simulink model "BalancingRobot_backup"  (R2020a)
settings: Solver=ode23t  StartTime=0.0  StopTime=20  RelTol=1e-2  EnableMultiTasking=on
values from neighbouring files (symbols this model uses):
  height_plane = 0.01    [DDPG_episdoe_508_maxtorque_2175e-01_Tf_10_Ts_1e-01_6DOF.mat]    (also in DDPG_episode_119_before_6dof_change_Ts_1e-01.mat)
  init_height = 0.109    [DDPG_episdoe_508_maxtorque_2175e-01_Tf_10_Ts_1e-01_6DOF.mat]    (also in DDPG_episode_119_before_6dof_change_Ts_1e-01.mat)
  max_torque = 0.2157463    [DDPG_episdoe_508_maxtorque_2175e-01_Tf_10_Ts_1e-01_6DOF.mat]    (also in DDPG_episode_119_before_6dof_change_Ts_1e-01.mat)
  plane_x = 10    [DDPG_episdoe_508_maxtorque_2175e-01_Tf_10_Ts_1e-01_6DOF.mat]    (also in DDPG_episode_119_before_6dof_change_Ts_1e-01.mat)
  plane_y = 1    [DDPG_episdoe_508_maxtorque_2175e-01_Tf_10_Ts_1e-01_6DOF.mat]    (also in DDPG_episode_119_before_6dof_change_Ts_1e-01.mat)
  table =     [DDPG_episdoe_508_maxtorque_2175e-01_Tf_10_Ts_1e-01_6DOF.mat]    (also in DDPG_episode_119_before_6dof_change_Ts_1e-01.mat)
  Tf = 10    [DDPG_episdoe_508_maxtorque_2175e-01_Tf_10_Ts_1e-01_6DOF.mat]    (also in DDPG_episode_119_before_6dof_change_Ts_1e-01.mat)
  Ts = 0.1    [DDPG_episdoe_508_maxtorque_2175e-01_Tf_10_Ts_1e-01_6DOF.mat]    (also in DDPG_episode_119_before_6dof_change_Ts_1e-01.mat)
  vx0 = 0    [DDPG_episdoe_508_maxtorque_2175e-01_Tf_10_Ts_1e-01_6DOF.mat]    (also in DDPG_episode_119_before_6dof_change_Ts_1e-01.mat)
  whl =     [DDPG_episdoe_508_maxtorque_2175e-01_Tf_10_Ts_1e-01_6DOF.mat]    (also in DDPG_episode_119_before_6dof_change_Ts_1e-01.mat)
undefined symbols (not defined in the file or in its folder): X, Y, Z
libraries: sm_lib x72, nesl_utility x22, Contact_Forces_Lib x14, simulink x8, rllib x1
(part 1 of 4)
settings Model: Creator=The MathWorks, Inc.  LastModifiedBy=User
settings SolverCC: ZeroCrossAlgorithm=Adaptive
settings DataIOCC: SaveOutput=off  SignalLogging=off  DSMLogging=off  SaveTime=off  ReturnWorkspaceOutputs=off  OutputTimes=0:0.01:10
settings OptimizationCC: LifeSpan=inf
settings DebuggingCC: MaxConsecutiveZCsMsg=warning  IgnoredZcDiagnostic=none  AllowSymbolicDim=off  SFUnexpectedBacktrackingDiag=warning  SFNoUnconditionalDefaultTransitionDiag=warning  SFExecutionAtInitializationDiag=none  UnitsInconsistencyMsg=none  ArithmeticOperatorsInVariantConditions=warning
settings SFSimCC: SimUseLocalCustomCode=off  CustomCodeUndefinedFunction=UseInterfaceOnly
settings RTWCC: RTWUseLocalCustomCode=off
settings CodeAppCC: StateflowObjectComments=on
settings GRTTargetCC: TargetLangStandard=C89/C90 (ANSI)
settings ConfigComp: CovMetricSettings=dw  CovHtmlReporting=on  CovSaveCumulativeToWorkspaceVar=on  CovSaveSingleToWorkspaceVar=on  CovExternalEMLEnable=off  CovSFcnEnable=off
settings SimscapeCC: SimscapeNormalizeSystem=off  SimscapeLogOpenViewer=on  SimscapeLogLimitData=off  SimscapeLogDataHistory=10000
settings ConfigurationSet: Description=SimMechanics 2G
settings DiagnosticsConfigSet: SimMechanicsRigidlyBoundBlock=none
settings ExplorerConfigSet: InternalSimMechanicsExplorerSettings="<ExplorerConfiguration><canonicalview>default</canonicalview><AnimationSetting><BasePlaybackSpeed>1.0</BasePlaybackSpeed><PlaybackSpeedFactor>1.0</PlaybackSpeedFactor></AnimationSetting><TilePanel><TileInfo><Tiles Columns=\"2\" Count=\"2\" Rows=\"1\"><Column Weight=\"0.5\"/><Column Weight=\"0.5\"/><Row Weight=\"1\"/><Tile Height=\"1\" Width=\"1\" X=\"0\" Y=\"0\"/><Tile Height=\"1\" Width=\"1\" X=\"1\" Y=\"0\"/></Tiles></TileInfo><SceneInfo><SceneViewer><BGColor><R>0.60000002384185791</R><G>0.60000002384185791</G><B>0.60000002384185791</B></BGColor><Camera><DoPerspective>on</DoPerspective><Position><X>1.10000000000000009</X><Y>0</Y><Z>0.200000000000000011</Z></Position><Center><X>0.0500000000000000028</X><Y>0.0899999999999999967</Y><Z>0.109</Z></Center><Up><X>0</X><Y>0</Y><Z>1</Z></Up><ViewLimDist>1</ViewLimDist><YLim>0.466307658154998583</YLim><XLim>0.322512345067554107</XLim></Camera></SceneViewer><SceneViewer><BGColor><R>0.60000002384185791</R><G>0.60000002384185791</G><B>0.60000002384185791</B></BGColor><Camera><DoPerspective>on</DoPerspective><Position><X>0.550000000000000044</X><Y>-0.570000000000000062</Y><Z>0.699999999999999956</Z></Position><Center><X>0.0500000000000000028</X><Y>0.0899999999999999967</Y><Z>0.109</Z></Center><Up><X>0</X><Y>0</Y><Z>1</Z></Up><ViewLimDist>1</ViewLimDist><YLim>0.466307658154998583</YLim><XLim>0.322512345067554107</XLim></Camera></SceneViewer></SceneInfo></TilePanel><MechEditorPanel><Cameras><Camera><Id>Camera1</Id><Value><Name>FrontView</Name><NativeCamera><PositionTrackingFeature>Walking_Robot.Camera.Front_View_Cam.F</PositionTrackingFeature><CenterTrackingFeature>Walking_Robot.Body.base</CenterTrackingFeature><UpVectorTrackingFeature>Walking_Robot.Body.base</UpVectorTrackingFeature><CenterTrackingOrigin>on</CenterTrackingOrigin><UpVectorTrackingDirection>+Z</UpVectorTrackingDirection></NativeCamera></Value></Camera><Camera><Id>Camera2</Id><Value><Name>sideView</Name><NativeCamera><PositionTrackingFeature>Walking_Robot.Camera.Side_View_Cam.F</PositionTrackingFeature><CenterTrackingFeature>Walking_Robot.Body.base</CenterTrackingFeature><UpVectorTrackingFeature>Walking_Robot.Body.base</UpVectorTrackingFeature><CenterTrackingOrigin>on</CenterTrackingOrigin><UpVectorTrackingDirection>+Z</UpVectorTrackingDirection></NativeCamera></Value></Camera></Cameras><GfxPanelCameraMap><MapElement CameraMLId=\"Camera1\" GfxPanelIndex=\"0\"/><MapElement CameraMLId=\"Camera2\" GfxPanelIndex=\"1\"/></GfxPanelCameraMap><VideoCreator><PlaybackSpeedRatio>1.0</PlaybackSpeedRatio><FrameRate>30</FrameRate><VideoFormat>Motion JPEG AVI</VideoFormat><FrameSize>auto</FrameSize></VideoCreator></MechEditorPanel></ExplorerConfiguration>"

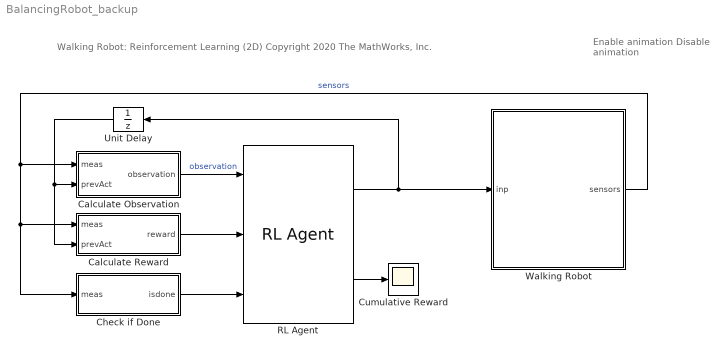
== system BalancingRobot_backup ==
  note: Enable animation
      |
      | Disable animation
  note: Walking Robot: Reinforcement Learning (2D)
      |
      | Copyright 2020 The MathWorks, Inc.
  Calculate Observation : Subsystem
  Calculate Reward : Subsystem
  Check if Done : Subsystem
  Cumulative Reward : Scope
  RL Agent : rllib/RL Agent  Agent=agent  ProvideReward=on  ProvideIsDone=on  ProvideCumRwd=on  TreatAsDirectFeedthrough=on  CollectLoggedSignals=on  CollectModelStates=on
  Unit Delay : UnitDelay  SampleTime=-1  HasFrameUpgradeWarning=on
  Walking Robot : Subsystem
  wires:
  Walking Robot/1(sensors) -> Check if Done/1(meas), Calculate Reward/1(meas), Calculate Observation/1(meas)  "sensors"
  Calculate Reward/1(reward) -> RL Agent/2
  Calculate Observation/1(observation) -> RL Agent/1  "observation"
  Check if Done/1(isdone) -> RL Agent/3
  RL Agent/2 -> Cumulative Reward/1
  Unit Delay/1 -> Calculate Reward/2(prevAct), Calculate Observation/2(prevAct)
  RL Agent/1 -> Walking Robot/1(inp), Unit Delay/1

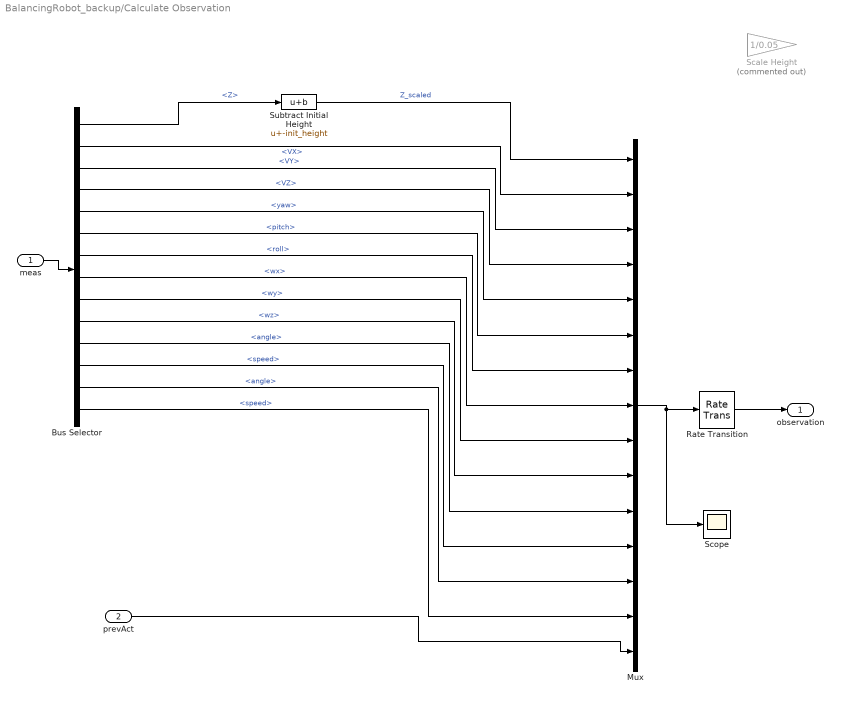
== system BalancingRobot_backup/Calculate Observation ==
  meas : Inport
  prevAct : Inport  Port=2
  Bus Selector : BusSelector  OutputSignals=Z,VX,VY,VZ,yaw,pitch,roll,wx,wy,wz,measL.angle,measL.speed,measR.angle,measR.speed
  Mux : Mux  Inputs=15
  Rate Transition : RateTransition
  Scale Height : Gain  Commented=on  Gain=1/0.05
  Scope : Scope
  Subtract Initial Height : Bias  Bias=-init_height
  observation : Outport  VectorParamsAs1DForOutWhenUnconnected=off
  wires:
  meas/1 -> Bus Selector/1
  Mux/1 -> Scope/1, Rate Transition/1
  Rate Transition/1 -> observation/1
  prevAct/1 -> Mux/15
  Bus Selector/1 -> Subtract Initial Height/1  "<Z>"
  Subtract Initial Height/1 -> Mux/1  "Z_scaled"
  Bus Selector/3 -> Mux/3  "<VY>"
  Bus Selector/4 -> Mux/4  "<VZ>"
  Bus Selector/2 -> Mux/2  "<VX>"
  Bus Selector/5 -> Mux/5  "<yaw>"
  Bus Selector/6 -> Mux/6  "<pitch>"
  Bus Selector/7 -> Mux/7  "<roll>"
  Bus Selector/8 -> Mux/8  "<wx>"
  Bus Selector/9 -> Mux/9  "<wy>"
  Bus Selector/10 -> Mux/10  "<wz>"
  Bus Selector/11 -> Mux/11  "<angle>"
  Bus Selector/12 -> Mux/12  "<speed>"
  Bus Selector/13 -> Mux/13  "<angle>"
  Bus Selector/14 -> Mux/14  "<speed>"

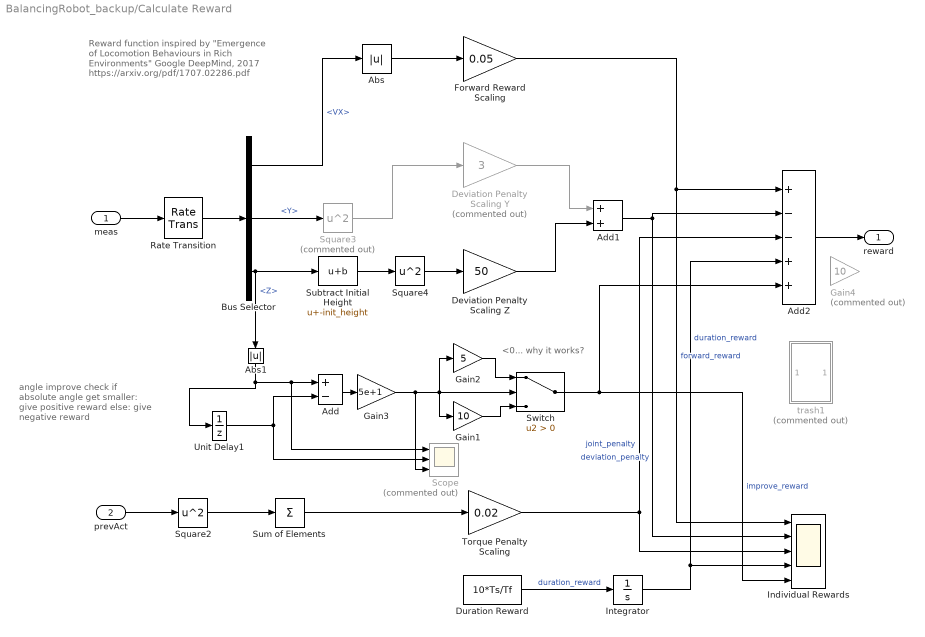
== system BalancingRobot_backup/Calculate Reward ==
  note: <0... why it works?
  note: angle improve check
      | if absolute angle get smaller:
      | 	give positive reward
      | else:
      | 	give negative reward
  note: Reward function inspired by
      | "Emergence of Locomotion Behaviours in Rich Environments"
      | Google DeepMind, 2017
      | https://arxiv.org/pdf/1707.02286.pdf
  meas : Inport
  prevAct : Inport  Port=2
  Abs : Abs
  Abs1 : Abs
  Add : Sum  Inputs=+-
  Add1 : Sum
  Add2 : Sum  Inputs=+--++
  Bus Selector : BusSelector  OutputSignals=VX,Y,Z
  Deviation Penalty Scaling Y : Gain  Commented=on  Gain=3
  Deviation Penalty Scaling Z : Gain  Gain=50
  Duration Reward : Constant  Value=10*Ts/Tf
  Forward Reward Scaling : Gain  Gain=0.05
  Gain1 : Gain  Gain=10
  Gain2 : Gain  Gain=5
  Gain3 : Gain  Gain=5e+1
  Gain4 : Gain  Commented=on  Gain=10
  Individual Rewards : Scope  NumInputPorts=5
  Integrator : Integrator
  Rate Transition : RateTransition  OutPortSampleTime=Ts
  Scope : Scope  Commented=on  NumInputPorts=3
  Square2 : Math  Operator=square  SignedPower=on  SaturateOnIntegerOverflow=on
  Square3 : Math  Commented=on  Operator=square  SignedPower=on  SaturateOnIntegerOverflow=on
  Square4 : Math  Operator=square  SignedPower=on  SaturateOnIntegerOverflow=on
  Subtract Initial Height : Bias  Bias=-init_height
  Sum of Elements : Sum  Inputs=+
  Switch : Switch  Criteria=u2 > Threshold
  Torque Penalty Scaling : Gain  Gain=0.02
  Unit Delay1 : UnitDelay  InitialCondition=init_height  SampleTime=Ts  HasFrameUpgradeWarning=on
  trash1 : Subsystem  Commented=on
  reward : Outport  VectorParamsAs1DForOutWhenUnconnected=off
  wires:
  meas/1 -> Rate Transition/1
  Rate Transition/1 -> Bus Selector/1
  Add2/1 -> reward/1
  Add1/1 -> Add2/2, Individual Rewards/2  "deviation_penalty"
  Forward Reward Scaling/1 -> Add2/1, Individual Rewards/1  "forward_reward"
  Sum of Elements/1 -> Torque Penalty Scaling/1
  Bus Selector/1 -> Abs/1  "<VX>"
  Square3/1 -> Deviation Penalty Scaling Y/1
  Duration Reward/1 -> Integrator/1  "duration_reward"
  prevAct/1 -> Square2/1
  Square2/1 -> Sum of Elements/1
  Torque Penalty Scaling/1 -> Add2/3, Individual Rewards/3  "joint_penalty"
  Square4/1 -> Deviation Penalty Scaling Z/1
  Bus Selector/3 -> Abs1/1, Subtract Initial Height/1  "<Z>"
  Subtract Initial Height/1 -> Square4/1
  Deviation Penalty Scaling Z/1 -> Add1/2
  Deviation Penalty Scaling Y/1 -> Add1/1
  Bus Selector/2 -> Square3/1  "<Y>"
  Abs/1 -> Forward Reward Scaling/1
  Unit Delay1/1 -> Scope/2, Add/2
  Gain1/1 -> Switch/3
  Gain2/1 -> Switch/1
  Switch/1 -> Individual Rewards/5, Add2/5  "improve_reward"
  Abs1/1 -> Unit Delay1/1, Scope/1, Add/1
  Add/1 -> Gain3/1
  Gain3/1 -> Scope/3, Gain1/1, Gain2/1, Switch/2
  Integrator/1 -> Add2/4, Individual Rewards/4  "duration_reward"

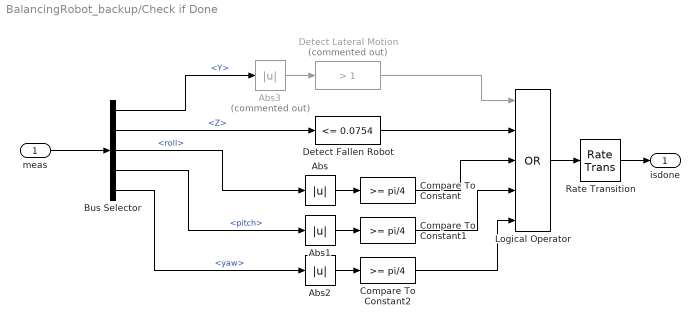
== system BalancingRobot_backup/Check if Done ==
  meas : Inport
  Abs : Abs
  Abs1 : Abs
  Abs2 : Abs
  Abs3 : Abs  Commented=on
  Bus Selector : BusSelector  OutputSignals=Y,Z,roll,pitch,yaw
  Compare To Constant : simulink/Logic and Bit Operations/Compare To Constant  relop=>=  const=pi/4  OutDataTypeStr=boolean
  Compare To Constant1 : simulink/Logic and Bit Operations/Compare To Constant  relop=>=  const=pi/4  OutDataTypeStr=boolean
  Compare To Constant2 : simulink/Logic and Bit Operations/Compare To Constant  relop=>=  const=pi/4  OutDataTypeStr=boolean
  Detect Fallen Robot : simulink/Logic and Bit Operations/Compare To Constant  relop=<=  const=0.0754  OutDataTypeStr=boolean
  Detect Lateral Motion : simulink/Logic and Bit Operations/Compare To Constant  Commented=on  relop=>  const=1  OutDataTypeStr=boolean
  Logical Operator : Logic  Operator=OR  Inputs=5  AllPortsSameDT=off  OutDataTypeStr=boolean
  Rate Transition : RateTransition
  isdone : Outport  VectorParamsAs1DForOutWhenUnconnected=off
  wires:
  Logical Operator/1 -> Rate Transition/1
  Bus Selector/2 -> Detect Fallen Robot/1  "<Z>"
  meas/1 -> Bus Selector/1
  Detect Fallen Robot/1 -> Logical Operator/2
  Bus Selector/3 -> Abs/1  "<roll>"
  Bus Selector/4 -> Abs1/1  "<pitch>"
  Compare To Constant/1 -> Logical Operator/3
  Abs/1 -> Compare To Constant/1
  Abs1/1 -> Compare To Constant1/1
  Compare To Constant1/1 -> Logical Operator/4
  Rate Transition/1 -> isdone/1
  Abs2/1 -> Compare To Constant2/1
  Bus Selector/5 -> Abs2/1  "<yaw>"
  Compare To Constant2/1 -> Logical Operator/5
  Abs3/1 -> Detect Lateral Motion/1
  Bus Selector/1 -> Abs3/1  "<Y>"
  Detect Lateral Motion/1 -> Logical Operator/1
